simulink model "KanKimMiy91_r2"  (R2018a)
settings: Solver=ode45  StartTime=0.0  StopTime=2  RelTol=1e-5  EnableMultiTasking=on
libraries: simulink x1
settings Model: Creator=dwbertol  LastModifiedBy=bruno
settings DataIOCC: LimitDataPoints=on  SaveFormat=Array  SignalLoggingSaveFormat=ModelDataLogs
settings OptimizationCC: ExpressionDepthLimit=2147483647  LifeSpan=inf
settings DebuggingCC: UnderspecifiedInitializationDetection=Classic  MergeDetectMultiDrivingBlocksExec=none  SolverPrmCheckMsg=warning  FcnCallInpInsideContextMsg=warning  StateNameClashWarn=warning  SFUnexpectedBacktrackingDiag=warning  SFNoUnconditionalDefaultTransitionDiag=warning  SFExecutionAtInitializationDiag=none
settings HardwareCC: ProdBitPerPointer=32  ProdBitPerSizeT=32  ProdBitPerPtrDiffT=32  ProdLargestAtomicFloat=None  ProdIntDivRoundTo=Undefined  ProdEndianess=Unspecified  ProdWordSize=32  ProdHWDeviceType=32-bit Generic
settings ModelReferenceCC: PropagateSignalLabelsOutOfModel=off
settings CodeAppCC: StateflowObjectComments=on
settings GRTTargetCC: TargetLangStandard=C89/C90 (ANSI)  GeneratePreprocessorConditionals=Disable all  CombineOutputUpdateFcns=off  GRTInterface=on
settings ConfigComp: CovMetricSettings=dw  CovHtmlReporting=on  CovSaveCumulativeToWorkspaceVar=on  CovSaveSingleToWorkspaceVar=on  CovExternalEMLEnable=off

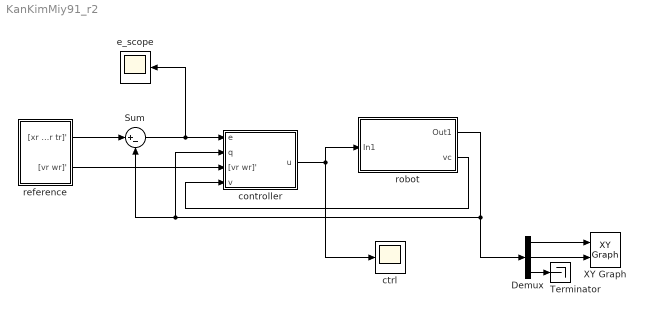
== system KanKimMiy91_r2 ==
  Demux : Demux  Outputs=3
  Sum : Sum  Inputs=|+-  AccumDataTypeStr=double
  Terminator : Terminator
  XY Graph : simulink/Sinks/XY Graph  xmin=-0.1  xmax=10  ymin=-0.1  ymax=10  st=-1
  controller : Subsystem  mask{kx=80, ky=284, kt=32, k4=2}
  ctrl : Scope
  e_scope : Scope
  reference : Subsystem  mask{vr=5, wr=0, ini=[0 6 0]}
  robot : Subsystem  mask{ini=[0 7 0]'}
  wires:
  controller/1(u) -> robot/1(In1), ctrl/1
  Demux/3 -> Terminator/1
  Demux/2 -> XY Graph/2
  Demux/1 -> XY Graph/1
  reference/1("[xr yr tr]' ") -> Sum/1
  Sum/1 -> e_scope/1, controller/1(e)
  reference/2("[vr wr]'") -> controller/3("[vr wr]'")
  robot/1(Out1) -> Demux/1, Sum/2, controller/2(q)
  robot/2(vc) -> controller/4(v)

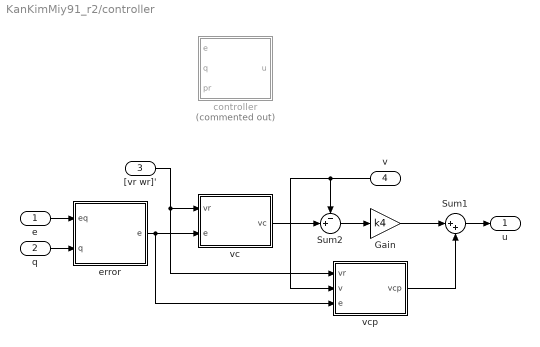
== system KanKimMiy91_r2/controller ==
  e : Inport
  q : Inport  Port=2
  "[vr wr]'" : Inport  Port=3
  v : Inport  Port=4
  Gain : Gain  Gain=k4
  Sum1 : Sum  Inputs=|++  AccumDataTypeStr=double
  Sum2 : Sum  Inputs=-+|  AccumDataTypeStr=double
  controller : MATLAB Function  Commented=on  TreatAsAtomicUnit=on
  error : MATLAB Function  TreatAsAtomicUnit=on
  vc : MATLAB Function  TreatAsAtomicUnit=on
  vcp : MATLAB Function  TreatAsAtomicUnit=on
  u : Outport
  wires:
  q/1 -> error/2(q)
  Gain/1 -> Sum1/1
  Sum2/1 -> Gain/1
  vcp/1(vcp) -> Sum1/2
  "[vr wr]'"/1 -> vc/1(vr), vcp/1(vr)
  error/1(e) -> vcp/3(e), vc/2(e)
  Sum1/1 -> u/1
  vc/1(vc) -> Sum2/2
  v/1 -> vcp/2(v), Sum2/1
  e/1 -> error/1(eq)

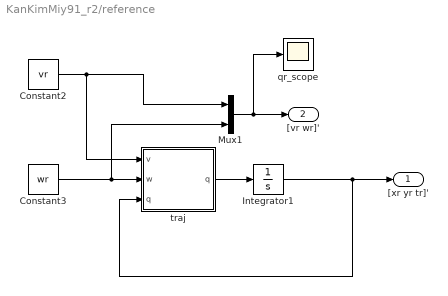
== system KanKimMiy91_r2/reference ==
  Constant2 : Constant  Value=vr  VectorParams1D=off
  Constant3 : Constant  Value=wr  VectorParams1D=off
  Integrator1 : Integrator  InitialCondition=ini
  Mux1 : Mux  Inputs=2
  qr_scope : Scope
  traj : MATLAB Function  TreatAsAtomicUnit=on
  "[xr yr tr]' " : Outport
  "[vr wr]'" : Outport  Port=2
  wires:
  Constant2/1 -> traj/1(v), Mux1/1
  Mux1/1 -> "[vr wr]'"/1, qr_scope/1
  traj/1(q) -> Integrator1/1
  Integrator1/1 -> "[xr yr tr]' "/1, traj/3("q ")
  Constant3/1 -> Mux1/2, traj/2(w)

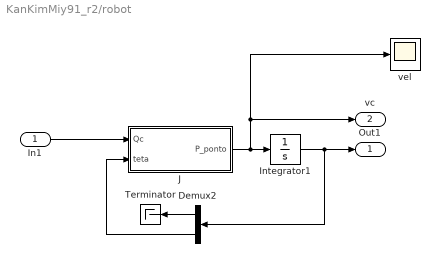
== system KanKimMiy91_r2/robot ==
  In1 : Inport
  Demux2 : Demux  Outputs=[2 1]
  Integrator1 : Integrator  InitialCondition=ini
  J : Subsystem
  Terminator : Terminator
  vel : Scope
  Out1 : Outport
  vc : Outport  Port=2
  wires:
  J/1(P_ponto) -> vc/1, vel/1, Integrator1/1
  Integrator1/1 -> Demux2/1, Out1/1
  Demux2/2 -> J/2(teta)
  Demux2/1 -> Terminator/1
  In1/1 -> J/1(Qc)

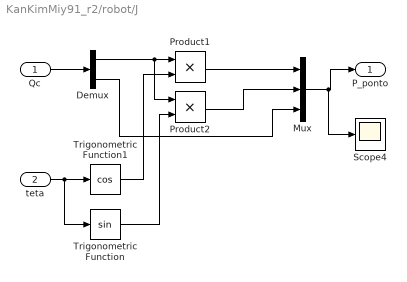
== system KanKimMiy91_r2/robot/J ==
  Qc : Inport
  teta : Inport  Port=2
  Demux : Demux  Outputs=2
  Mux : Mux  Inputs=3
  Product1 : Product
  Product2 : Product
  Scope4 : Scope
  Trigonometric Function : Trigonometry
  Trigonometric Function1 : Trigonometry  Operator=cos
  P_ponto : Outport
  wires:
  Mux/1 -> Scope4/1, P_ponto/1
  Qc/1 -> Demux/1
  teta/1 -> Trigonometric Function/1, Trigonometric Function1/1
  Trigonometric Function1/1 -> Product1/2
  Demux/1 -> Product2/1, Product1/1
  Product1/1 -> Mux/1
  Trigonometric Function/1 -> Product2/2
  Product2/1 -> Mux/2
  Demux/2 -> Mux/3

== matlab function KanKimMiy91_r2/reference/traj ==
  data: v input; w input; q input; q output
function q = fcn(v, w, q)

 q = [cos(q(3)) 0; sin(q(3)) 0; 0 1]*[v; w];
 
end

== matlab function KanKimMiy91_r2/controller/error ==
  data: eq input; e output; q input
function e = fcn(eq,q)
%#eml

 Te = [cos(q(3)) sin(q(3)) 0; -sin(q(3)) cos(q(3)) 0; 0 0 1];
 
 e = Te*eq;

end

== matlab function KanKimMiy91_r2/controller/vc ==
  data: vr input; e input; vc output; kx parameter; ky parameter; kt parameter
function vc = fcn(vr,e,kx,ky,kt)
%#eml


 vc = [vr(1)*cos(e(3))+kx*e(1);vr(2)+ky*vr(1)*e(2)+kt*vr(1)*sin(e(3))];
 
end

== matlab function KanKimMiy91_r2/controller/controller ==
  data: e input; q input; pr input; u output; kx parameter; ky parameter; kt parameter
function u = fcn(e,q,pr,kx,ky,kt)

 pe = [cos(q(3)) sin(q(3)) 0; -sin(q(3)) cos(q(3)) 0; 0 0 1]*e;

 u = [pr(1)*cos(pe(3))+kx*pe(1) pr(2)+pr(1)*(ky*pe(2)+kt*sin(pe(3)))]';
 
end

== matlab function KanKimMiy91_r2/controller/vcp ==
  data: vr input; v input; e input; vcp output; kx parameter; ky parameter; kt parameter
function vcp = fcn(vr,v,e,kx,ky,kt)
%#eml

 ep = [v(2)*e(2)-v(1)+vr(1)*cos(e(3));-v(2)*e(1)+vr(1)*sin(e(3));vr(2)-v(2)];
 vcp = [kx 0 -vr(1)*sin(e(3)); 0 ky*vr(1) kt*vr(1)*cos(e(3))]*ep;
 
end
